simulink model "AttitudeDynamics"  (R2018b)
settings: configuration reference "RPi_DynamicsRate" (kept outside this file)
InitFcn:
  | loadThrusterData
undefined symbols (not defined in the file or in its folder): DiscIntNeverNeededParam
settings Model: Creator=Andy  LastModifiedBy=barthal
settings ConfigSetRef: SourceLocation=Base Workspace

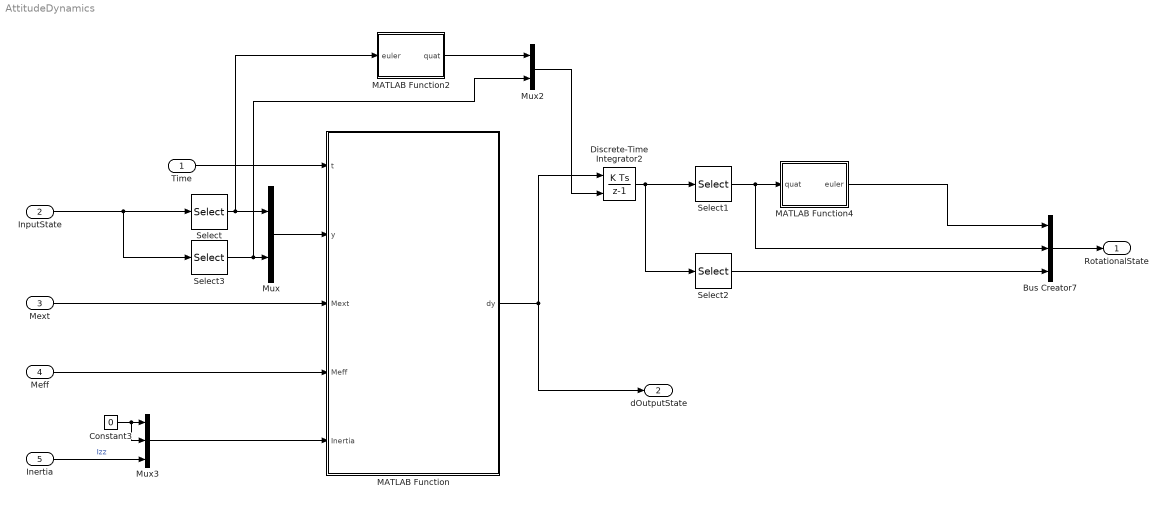
== system AttitudeDynamics ==
  Time : Inport  OutDataTypeStr=double  PortDimensions=1
  InputState : Inport  Port=2  OutDataTypeStr=double
  Mext : Inport  Port=3  OutDataTypeStr=double  PortDimensions=3
  Meff : Inport  Port=4  OutDataTypeStr=double  PortDimensions=3
  Inertia : Inport  Port=5  OutDataTypeStr=double  PortDimensions=1
  Bus Creator7 : BusCreator  Inputs=3  OutDataTypeStr=Bus: RotStateBodyECEFBus
      settings: InheritFromInputs=off
  Constant3 : Constant  Value=0
  Discrete-Time Integrator2 : DiscreteIntegrator  InitialConditionSource=external  SampleTime=-1  ICPrevOutput=DiscIntNeverNeededParam  ICPrevScaledInput=DiscIntNeverNeededParam
  MATLAB Function : MATLAB Function  TreatAsAtomicUnit=on
  MATLAB Function2 : MATLAB Function  TreatAsAtomicUnit=on
  MATLAB Function4 : MATLAB Function  TreatAsAtomicUnit=on
  Mux : Mux  Inputs=2
  Mux2 : Mux  Inputs=2
  Mux3 : Mux  Inputs=3
  Select : Selector  InputPortWidth=6  IndexOptions=Index vector (dialog)  Indices=[1:3]  OutputSizes=1
  Select1 : Selector  InputPortWidth=7  IndexOptions=Index vector (dialog)  Indices=[1:4]  OutputSizes=1
  Select2 : Selector  InputPortWidth=7  IndexOptions=Index vector (dialog)  Indices=[5:7]  OutputSizes=1
  Select3 : Selector  InputPortWidth=6  IndexOptions=Index vector (dialog)  Indices=[4:6]  OutputSizes=1
  RotationalState : Outport  OutDataTypeStr=Bus: RotStateBodyECEFBus
  dOutputState : Outport  Port=2  OutDataTypeStr=double
  wires:
  Time/1 -> MATLAB Function/1(t)
  InputState/1 -> Select3/1, Select/1
  Mux/1 -> MATLAB Function/2(y)
  Mext/1 -> MATLAB Function/3(Mext)
  Constant3/1 -> Mux3/2, Mux3/1
  Inertia/1 -> Mux3/3  "Izz"
  Mux3/1 -> MATLAB Function/5(Inertia)
  Select/1 -> Mux/1, MATLAB Function2/1(euler)
  Select3/1 -> Mux/2, Mux2/2
  Meff/1 -> MATLAB Function/4(Meff)
  MATLAB Function2/1(quat) -> Mux2/1
  MATLAB Function/1(dy) -> dOutputState/1, Discrete-Time Integrator2/1
  Select1/1 -> Bus Creator7/2, MATLAB Function4/1(quat)
  Discrete-Time Integrator2/1 -> Select1/1, Select2/1
  Mux2/1 -> Discrete-Time Integrator2/2
  MATLAB Function4/1(euler) -> Bus Creator7/1
  Bus Creator7/1 -> RotationalState/1
  Select2/1 -> Bus Creator7/3

== matlab function AttitudeDynamics/MATLAB Function ==
  data: t input; dy output; y input; Mext input; Meff input; Inertia input
function dy  = callrotationalEOM(t,y,Mext,Meff,Inertia)

 [dy] = rotationalEOM(t,y,Mext,Meff,Inertia);

== matlab function AttitudeDynamics/MATLAB Function2 ==
  data: euler input; quat output
function quat = fcn(euler)
quat = euler2quat(euler);

== matlab function AttitudeDynamics/MATLAB Function4 ==
  data: quat input; euler output
function euler = fcn(quat)

euler = quat2euler(quat');
